simulink library "pll_lib"  (Simulink 6.6)
libraries: simulink x4, pll_lib x2
settings Model: Creator=pluto  LastModifiedBy=kumm  ExtModeAutoUpdateStatusClock=off

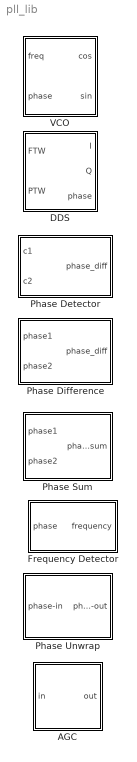
== system pll_lib ==
  AGC : Subsystem  TreatAsAtomicUnit=on  mask{Ts=10E-9, target_amplitude=1, agc_gain=100, agc_bandwidth=10E3}
      mask prompts: Ts "Sample Time"; target_amplitude "Target Amplitude"; agc_gain "AGC Gain"; agc_bandwidth "AGC bandwidth"
  DDS : Subsystem  TreatAsAtomicUnit=on  mask{wordlength=16, sampletime=-1}
      mask prompts: sampletime "sample time (-1 for inherited)"
      mask help:
      | Direct Digital Synthesizer
      | Output-Frequency and -Phase are defined as follows:
      | f_o=FTW/2^Wordlength*f_s
      | phase_o=Phase-Word/2^Wordlength*2*pi
      | f_s=1/T_s (Sample Frequency)
  Frequency Detector : Subsystem  TreatAsAtomicUnit=on  mask{Ts=10E-9}
      mask prompts: Ts "Sample Time"
      mask help: This block calculates the instantaneous frequency value in Hz of a given phase signal.
  Phase Detector : Subsystem  TreatAsAtomicUnit=on
      mask Description:
      | Calculates the phase difference from the two complex input signals c1 and c2 (arg(c1)-arg(c2)).
      | The phase difference is modulus 2*pi - pi (fittet in the range -pi...pi)
  Phase Difference : Subsystem  TreatAsAtomicUnit=on
      mask Description:
      | This block calculates a phase difference from the two inputs (phase1-phase2)
      | The phase difference is modulus 2*pi-pi (fittet in the range -pi...pi)
  Phase Sum : Subsystem  TreatAsAtomicUnit=on
      mask Description:
      | This block calculates a phase sum from the two inputs (phase1+phase2)
      | The phase sum is modulus 2*pi-pi (fittet in the range -pi...pi)
  Phase Unwrap : Subsystem  TreatAsAtomicUnit=on  mask{N=100}
      mask prompts: N "No. of periods to unwrap"
      mask help: Phase Unwrapper is similar than the matlap phase_unwrap function. A input signal in the range -pi...pi is unwrapped at every phase step of larger than 0.8*2*pi.
  VCO : Subsystem  Description=Voltage Controlled Oscillator  TreatAsAtomicUnit=on  mask{init_phase=0}
      mask prompts: init_phase "init phase"
      mask help:
      | Voltage Controled Oscilator
      | f_out=freq_in in Hz
      | K0=2*pi
      mask Help: Outputs are I (cos) and Q (sin) Phase

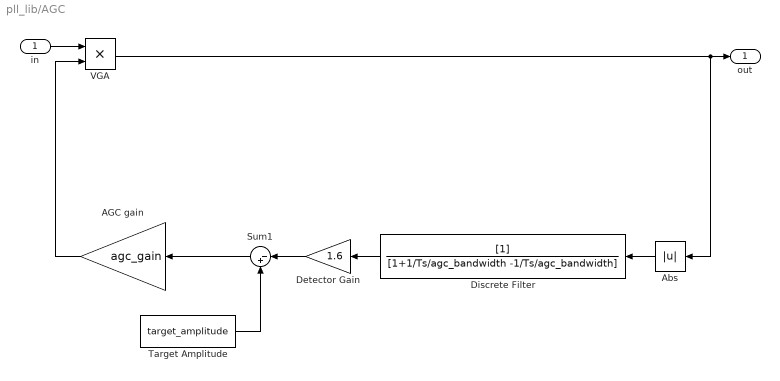
== system pll_lib/AGC ==
  in : Inport
  AGC gain : Gain  Orientation=left  Gain=agc_gain
  Abs : Abs  Orientation=left
  Detector Gain : Gain  Orientation=left  Gain=1.6
  Discrete Filter : DiscreteFilter  Orientation=left  Denominator=[1+1/Ts/agc_bandwidth -1/Ts/agc_bandwidth]  SampleTime=Ts
  Sum1 : Sum  Orientation=left  Inputs=|-+
  Target Amplitude : Constant  Value=target_amplitude
  VGA : Product  RndMeth=Zero
  out : Outport
  wires:
  VGA/1 -> out/1, Abs/1
  Target Amplitude/1 -> Sum1/2
  AGC gain/1 -> VGA/2
  Sum1/1 -> AGC gain/1
  in/1 -> VGA/1
  Abs/1 -> Discrete Filter/1
  Discrete Filter/1 -> Detector Gain/1
  Detector Gain/1 -> Sum1/1

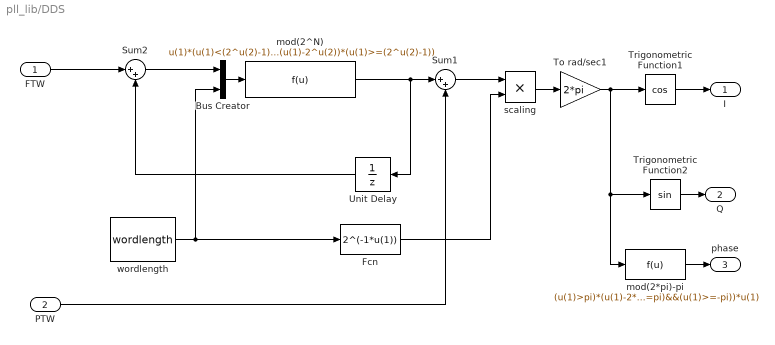
== system pll_lib/DDS ==
  FTW : Inport
  PTW : Inport  Port=2
  Bus Creator : BusCreator  Inputs=2
  Fcn : Fcn  Expr=2^(-1*u(1))  SampleTime=sampletime
  Sum1 : Sum  Inputs=|++  SampleTime=sampletime
  Sum2 : Sum  Inputs=|++  SampleTime=sampletime
  To rad/sec1 : Gain  Gain=2*pi  SampleTime=sampletime
  Trigonometric Function1 : Trigonometry  Operator=cos  SampleTime=sampletime
  Trigonometric Function2 : Trigonometry  SampleTime=sampletime
  Unit Delay : UnitDelay  Orientation=left  SampleTime=sampletime
  mod(2*pi)-pi : Fcn  Expr=(u(1)>pi)*(u(1)-2*pi)+(u(1)<-pi)*(u(1)+2*pi)+((u(1)<=pi)&&(u(1)>=-pi))*u(1)
  mod(2^N) : Fcn  Expr=u(1)*(u(1)<(2^u(2)-1))+(u(1)-2^u(2))*(u(1)>=(2^u(2)-1))  SampleTime=sampletime
  scaling : Product  SampleTime=sampletime  RndMeth=Zero
  wordlength : Constant  Value=wordlength  SampleTime=sampletime
  I : Outport
  Q : Outport  Port=2
  phase : Outport  Port=3
  wires:
  To rad/sec1/1 -> Trigonometric Function1/1, Trigonometric Function2/1, mod(2*pi)-pi/1
  mod(2^N)/1 -> Sum1/1, Unit Delay/1
  FTW/1 -> Sum2/1
  Trigonometric Function2/1 -> Q/1
  wordlength/1 -> Fcn/1, Bus Creator/2
  Trigonometric Function1/1 -> I/1
  scaling/1 -> To rad/sec1/1
  Sum1/1 -> scaling/1
  PTW/1 -> Sum1/2
  Unit Delay/1 -> Sum2/2
  Fcn/1 -> scaling/2
  Bus Creator/1 -> mod(2^N)/1
  Sum2/1 -> Bus Creator/1
  mod(2*pi)-pi/1 -> phase/1

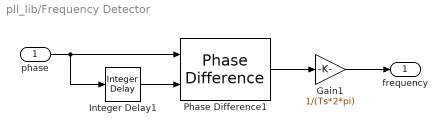
== system pll_lib/Frequency Detector ==
  phase : Inport
  Gain1 : Gain  Gain=1/(Ts*2*pi)  SampleTime=Ts
  Integer Delay1 : simulink/Discrete/Integer Delay  vinit=0.0  samptime=Ts  NumDelays=1
  Phase Difference1 : pll_lib/Phase Difference
  frequency : Outport
  wires:
  phase/1 -> Integer Delay1/1, Phase Difference1/1
  Integer Delay1/1 -> Phase Difference1/2
  Phase Difference1/1 -> Gain1/1
  Gain1/1 -> frequency/1

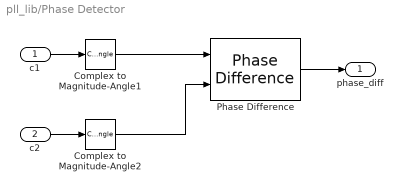
== system pll_lib/Phase Detector ==
  c1 : Inport
  c2 : Inport  Port=2
  Complex to Magnitude-Angle1 : ComplexToMagnitudeAngle  Output=Angle
  Complex to Magnitude-Angle2 : ComplexToMagnitudeAngle  Output=Angle
  Phase Difference : pll_lib/Phase Difference
  phase_diff : Outport
  wires:
  Complex to Magnitude-Angle1/1 -> Phase Difference/1
  Complex to Magnitude-Angle2/1 -> Phase Difference/2
  c1/1 -> Complex to Magnitude-Angle1/1
  c2/1 -> Complex to Magnitude-Angle2/1
  Phase Difference/1 -> phase_diff/1

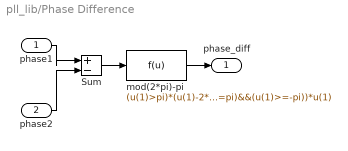
== system pll_lib/Phase Difference ==
  phase1 : Inport
  phase2 : Inport  Port=2
  Sum : Sum  Inputs=|+-
  mod(2*pi)-pi : Fcn  Expr=(u(1)>pi)*(u(1)-2*pi)+(u(1)<-pi)*(u(1)+2*pi)+((u(1)<=pi)&&(u(1)>=-pi))*u(1)
  phase_diff : Outport
  wires:
  Sum/1 -> mod(2*pi)-pi/1
  mod(2*pi)-pi/1 -> phase_diff/1
  phase1/1 -> Sum/1
  phase2/1 -> Sum/2

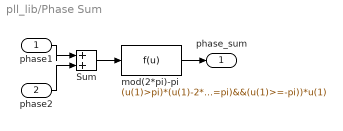
== system pll_lib/Phase Sum ==
  phase1 : Inport
  phase2 : Inport  Port=2
  Sum : Sum  Inputs=|++
  mod(2*pi)-pi : Fcn  Expr=(u(1)>pi)*(u(1)-2*pi)+(u(1)<-pi)*(u(1)+2*pi)+((u(1)<=pi)&&(u(1)>=-pi))*u(1)
  phase_sum : Outport
  wires:
  Sum/1 -> mod(2*pi)-pi/1
  phase1/1 -> Sum/1
  mod(2*pi)-pi/1 -> phase_sum/1
  phase2/1 -> Sum/2

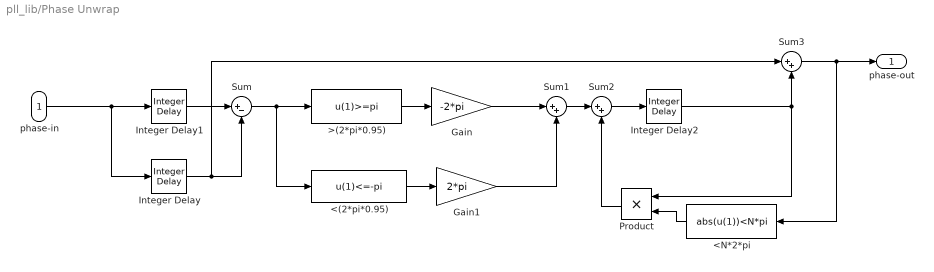
== system pll_lib/Phase Unwrap ==
  phase-in : Inport
  <(2*pi*0.95) : Fcn  Expr=u(1)<=-pi
  <N*2*pi : Fcn  Orientation=left  Expr=abs(u(1))<N*pi
  >(2*pi*0.95) : Fcn  Expr=u(1)>=pi
  Gain : Gain  Gain=-2*pi
  Gain1 : Gain  Gain=2*pi
  Integer Delay : simulink/Discrete/Integer Delay  vinit=0.0  samptime=-1  NumDelays=2
  Integer Delay1 : simulink/Discrete/Integer Delay  vinit=0.0  samptime=-1  NumDelays=1
  Integer Delay2 : simulink/Discrete/Integer Delay  vinit=0.0  samptime=-1  NumDelays=1
  Product : Product  Orientation=left  RndMeth=Zero
  Sum : Sum  Inputs=|+-
  Sum1 : Sum  Inputs=|++
  Sum2 : Sum  Inputs=|++
  Sum3 : Sum  Inputs=|++
  phase-out : Outport
  wires:
  Integer Delay/1 -> Sum/2, Sum3/1
  Sum/1 -> >(2*pi*0.95)/1, <(2*pi*0.95)/1
  <(2*pi*0.95)/1 -> Gain1/1
  >(2*pi*0.95)/1 -> Gain/1
  Integer Delay1/1 -> Sum/1
  Gain1/1 -> Sum1/2
  Gain/1 -> Sum1/1
  Sum1/1 -> Sum2/1
  Sum2/1 -> Integer Delay2/1
  Integer Delay2/1 -> Sum3/2, Product/1
  phase-in/1 -> Integer Delay/1, Integer Delay1/1
  Sum3/1 -> phase-out/1, <N*2*pi/1
  <N*2*pi/1 -> Product/2
  Product/1 -> Sum2/2

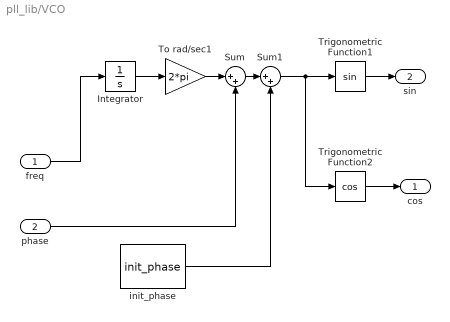
== system pll_lib/VCO ==
  freq : Inport  Description=Frequency in Hz
  phase : Inport  Port=2
  Integrator : Integrator
  Sum : Sum  Inputs=|++
  Sum1 : Sum  Inputs=|++
  To rad/sec1 : Gain  Gain=2*pi
  Trigonometric Function1 : Trigonometry
  Trigonometric Function2 : Trigonometry  Operator=cos
  init_phase : Constant  Value=init_phase
  cos : Outport
  sin : Outport  Port=2
  wires:
  Trigonometric Function2/1 -> cos/1
  freq/1 -> Integrator/1
  Trigonometric Function1/1 -> sin/1
  Integrator/1 -> To rad/sec1/1
  phase/1 -> Sum/2
  To rad/sec1/1 -> Sum/1
  Sum/1 -> Sum1/1
  Sum1/1 -> Trigonometric Function2/1, Trigonometric Function1/1
  init_phase/1 -> Sum1/2
